simulink model "pendulum"  (R2015b)
settings: Solver=FixedStepAuto  StartTime=0.0  StopTime=5  FixedStep=1/30  RelTol=1e-3
settings Model: Creator=Andreas  LastModifiedBy=Andreas

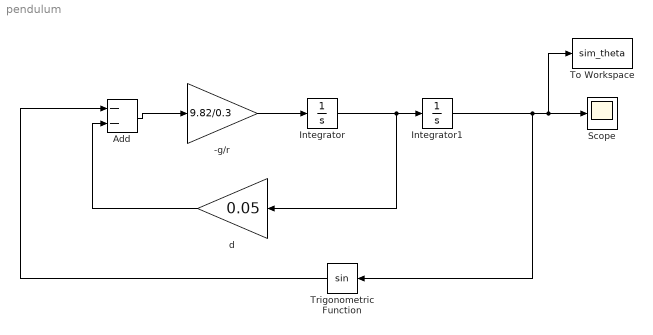
== system pendulum ==
  -g/r : Gain  Gain=9.82/0.3
  Add : Sum  Inputs=--
  Integrator : Integrator
  Integrator1 : Integrator  InitialCondition=1.5
  Scope : Scope
  To Workspace : ToWorkspace  VariableName=sim_theta  SaveFormat=Timeseries  SampleTime=-1
  Trigonometric Function : Trigonometry
  d : Gain  Gain=0.05
  wires:
  -g/r/1 -> Integrator/1
  Integrator1/1 -> Trigonometric Function/1, To Workspace/1, Scope/1
  Trigonometric Function/1 -> Add/1
  Add/1 -> -g/r/1
  Integrator/1 -> d/1, Integrator1/1
  d/1 -> Add/2
